simulink model "OpPointTest"  (R2024b)
settings: Solver=VariableStepAuto  StartTime=0.0  StopTime=60  FixedStep=0.02  RelTol=1e-3
values from neighbouring files (symbols this model uses):
  act_ailerons = 0    [OpPointTest_main.m]    (also in SG_model_trim.m = op.inputs(1).u; trim_op_fixed_v.mat)
  act_rear = 4    [OpPointTest_main.m]    (also in SG_model_trim.m = op.inputs(2).u; trim_op_fixed_v.mat = 2.35)
  initial_P = 0    [OpPointTest_main.m]    (also in SG_model_trim.m = op.states(4).x; trim_op_fixed_v.mat)
  initial_Pitch = -3.558    [OpPointTest_main.m]    (also in SG_model_trim.m = op.states(7).x; trim_op_fixed_v.mat = 0)
  initial_Q = 0    [OpPointTest_main.m]    (also in SG_model_trim.m = op.states(5).x; trim_op_fixed_v.mat)
  initial_R = 0    [OpPointTest_main.m]    (also in SG_model_trim.m = op.states(6).x; trim_op_fixed_v.mat)
  initial_ROLL = 0    [OpPointTest_main.m]    (also in SG_model_trim.m = op.states(8).x; trim_op_fixed_v.mat)
  initial_uspeed = cos(deg2rad(-3.558))*10.275    [OpPointTest_main.m]    (also in SG_model_trim.m = op.states(1).x; linear_model.mat = 10.285; trim_op_fixed_v.mat = 10.285)
  initial_vspeed = 0    [OpPointTest_main.m]    (also in SG_model_trim.m = op.states(2).x; trim_op_fixed_v.mat)
  initial_wspeed = sin(deg2rad(-3.558))*10.275    [OpPointTest_main.m]    (also in SG_model_trim.m = op.states(3).x; trim_op_fixed_v.mat = 0)
  initial_YAW = 0    [OpPointTest_main.m]    (also in SG_model_trim.m = op.states(9).x; trim_op_fixed_v.mat)
  initial_Z = 100    [OpPointTest_main.m]    (also in SG_model_trim.m = op.states(10).x; trim_op_fixed_v.mat = -50)
  T = 2679.2979205956    (= 2679.2979206)    [OpPointTest_main.m]    (also in SG01_Flight_Dynamics.m = rho*(Rpms_propeller/60)^2*diam^4*kt; SG01_Flight_Dynamics_original.m = rho*(Rpms_propeller/60)^2*diam^4*kt; SG_model_trim.m = op.inputs(3).u; trim_op_fixed_v.mat = 4651.4278561)
settings Model: Creator=Basile  LastModifiedBy=ricar
settings SolverCC: ConcurrentTasks=on  ZeroCrossAlgorithm=Adaptive  AlgebraicLoopSolver=TrustRegion  PositivePriorityOrder=on
settings DataIOCC: ExternalInput=getinputstruct(op_trim1)  InitialState=getstatestruct(op_trim1)  SaveOutput=off  DSMLogging=off  SaveTime=off  ReturnWorkspaceOutputs=off
settings OptimizationCC: BlockReduction=off  DefaultParameterBehavior=Inlined  UseDivisionForNetSlopeComputation=on  UseFloatMulNetSlope=on  OptimizeBlockIOStorage=off  BufferReuse=off  PassReuseOutputArgsThreshold=0  EfficientFloat2IntCast=on  OptimizeBlockOrder=speed  DifferentSizesBufferReuse=on
settings DebuggingCC: InheritedTsInSrcMsg=none  TasksWithSamePriorityMsg=none  ParameterTunabilityLossMsg=error  UniqueDataStoreMsg=error  ArithmeticOperatorsInVariantConditions=warning
settings HardwareCC: ProdBitPerLong=64  ProdLongLongMode=on  ProdHWDeviceType=Intel->x86-64 (Linux 64)
settings ModelReferenceCC: EnableRefExpFcnMdlSchedulingChecks=on
settings SFSimCC: SimUseLocalCustomCode=off  MATLABDynamicMemAlloc=off  CustomCodeUndefinedFunction=UseInterfaceOnly
settings RTWCC: Description=Simulink Real-Time  SystemTargetFile=slrealtime.tlc  TemplateMakefile=slrealtime_default_tmf  GenerateReport=on  RTWUseLocalCustomCode=off  Toolchain=Simulink Real-Time Toolchain  BuildConfiguration=Faster Runs  LaunchReport=on  CodeExecutionProfiling=on  TargetLang=C++  GPUComputeCapability=3.5  DLArmComputeVersion=19.05
settings CodeAppCC: ForceParamTrailComments=on  OperatorAnnotations=on
settings SimulinkRealTimeTargetCC: InstructionSetFMA=off  LogToMDFFile=off

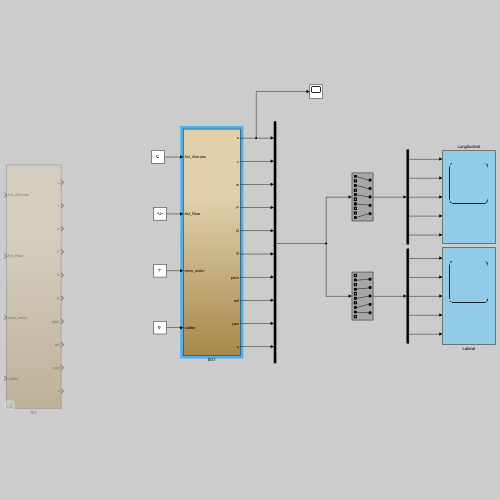
[thumbnail: Simulink's stored preview of the top-level diagram]
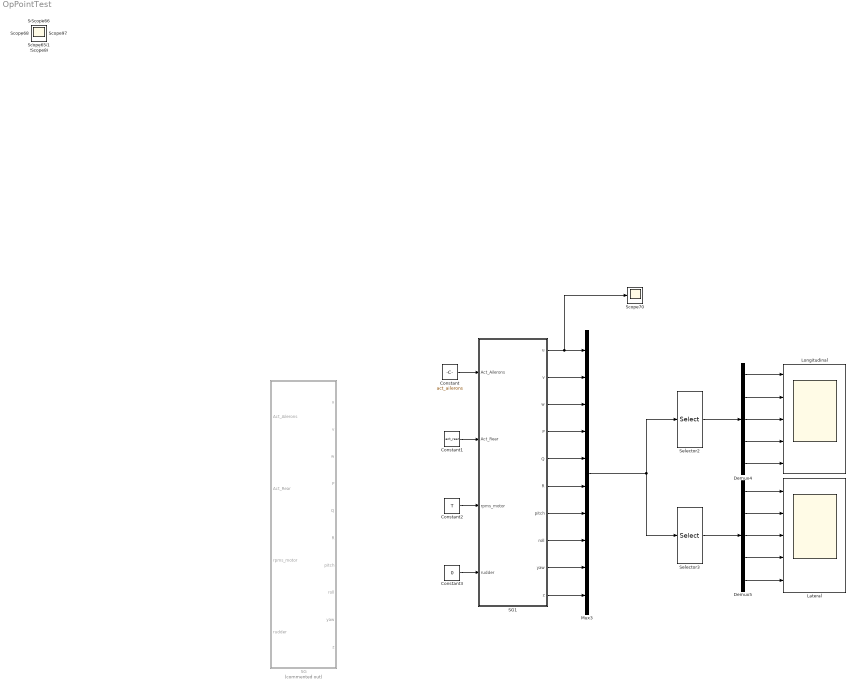
== system OpPointTest ==
  Constant : Constant  Value=act_ailerons
  Constant1 : Constant  Value=act_rear
  Constant2 : Constant  Value=T
  Constant3 : Constant  Value=0
  Demux4 : Demux  Outputs=5
  Demux5 : Demux  Outputs=5
  Lateral : Scope  NumInputPorts=5
  Longitudinal : Scope  NumInputPorts=5
  Mux3 : Mux  Inputs=10
  SG : Subsystem  Commented=on
  SG1 : Subsystem
  Scope{,1..68,70} (70 alike) : Scope
  Selector2 : Selector  InputPortWidth=10  IndexOptions=Index vector (dialog)  Indices=[1 3 5 7 10]  OutputSizes=1
  Selector3 : Selector  InputPortWidth=10  IndexOptions=Index vector (dialog)  Indices=[2 4 6 8 9]  OutputSizes=1
  wires:
  SG1/5(Q) -> Mux3/5
  SG1/6(R) -> Mux3/6
  SG1/7(pitch) -> Mux3/7
  SG1/10(z) -> Mux3/10
  SG1/4(P) -> Mux3/4
  SG1/8(roll) -> Mux3/8
  Demux5/3 -> Lateral/3
  Demux5/4 -> Lateral/4
  Selector2/1 -> Demux4/1
  Mux3/1 -> Selector2/1, Selector3/1
  Selector3/1 -> Demux5/1
  Demux5/2 -> Lateral/2
  Demux4/1 -> Longitudinal/1
  Demux5/5 -> Lateral/5
  Demux5/1 -> Lateral/1
  SG1/1(u) -> Scope70/1, Mux3/1
  SG1/9(yaw) -> Mux3/9
  Demux4/2 -> Longitudinal/2
  Demux4/4 -> Longitudinal/4
  Demux4/3 -> Longitudinal/3
  SG1/3(w) -> Mux3/3
  SG1/2(v) -> Mux3/2
  Demux4/5 -> Longitudinal/5
  Constant/1 -> SG1/1(Act_Ailerons)
  Constant1/1 -> SG1/2(Act_Rear)
  Constant2/1 -> SG1/3(rpms_motor)
  Constant3/1 -> SG1/4(rudder)

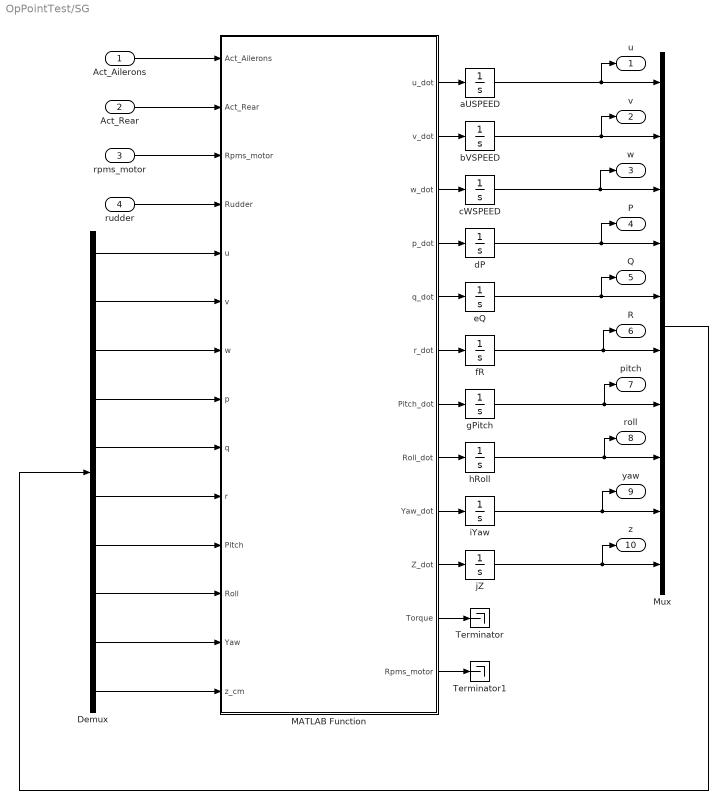
== system OpPointTest/SG ==
  Act_Ailerons : Inport
  Act_Rear : Inport  Port=2
  rpms_motor : Inport  Port=3
  rudder : Inport  Port=4
  Demux : Demux  Outputs=10
  MATLAB Function : MATLAB Function  TreatAsAtomicUnit=on
  Mux : Mux  Inputs=10
  Terminator : Terminator
  Terminator1 : Terminator
  aUSPEED : Integrator  InitialCondition=initial_uspeed
  bVSPEED : Integrator  InitialCondition=initial_vspeed
  cWSPEED : Integrator  InitialCondition=initial_wspeed
  dP : Integrator  InitialCondition=initial_P
  eQ : Integrator  InitialCondition=initial_Q
  fR : Integrator  InitialCondition=initial_R
  gPitch : Integrator  InitialCondition=initial_Pitch
  hRoll : Integrator  InitialCondition=initial_ROLL
  iYaw : Integrator  InitialCondition=initial_YAW
  jZ : Integrator  InitialCondition=initial_Z
  u : Outport
  v : Outport  Port=2
  w : Outport  Port=3
  P : Outport  Port=4
  Q : Outport  Port=5
  R : Outport  Port=6
  pitch : Outport  Port=7
  roll : Outport  Port=8
  yaw : Outport  Port=9
  z : Outport  Port=10
  wires:
  MATLAB Function/8(Roll_dot) -> hRoll/1
  Act_Rear/1 -> MATLAB Function/2(Act_Rear)
  rudder/1 -> MATLAB Function/4(Rudder)
  MATLAB Function/3(w_dot) -> cWSPEED/1
  Demux/3 -> MATLAB Function/7(w)
  MATLAB Function/11(Torque) -> Terminator/1
  MATLAB Function/6(r_dot) -> fR/1
  Demux/9 -> MATLAB Function/13(Yaw)
  Mux/1 -> Demux/1
  Demux/4 -> MATLAB Function/8(p)
  Demux/8 -> MATLAB Function/12(Roll)
  MATLAB Function/2(v_dot) -> bVSPEED/1
  Act_Ailerons/1 -> MATLAB Function/1(Act_Ailerons)
  MATLAB Function/1(u_dot) -> aUSPEED/1
  Demux/6 -> MATLAB Function/10(r)
  MATLAB Function/10(Z_dot) -> jZ/1
  rpms_motor/1 -> MATLAB Function/3("Rpms_motor ")
  MATLAB Function/12(Rpms_motor) -> Terminator1/1
  MATLAB Function/4(p_dot) -> dP/1
  Demux/1 -> MATLAB Function/5(u)
  MATLAB Function/9(Yaw_dot) -> iYaw/1
  Demux/7 -> MATLAB Function/11(Pitch)
  Demux/5 -> MATLAB Function/9(q)
  Demux/10 -> MATLAB Function/14(z_cm)
  MATLAB Function/7(Pitch_dot) -> gPitch/1
  MATLAB Function/5(q_dot) -> eQ/1
  Demux/2 -> MATLAB Function/6(v)
  aUSPEED/1 -> u/1, Mux/1
  bVSPEED/1 -> v/1, Mux/2
  cWSPEED/1 -> w/1, Mux/3
  dP/1 -> P/1, Mux/4
  eQ/1 -> Q/1, Mux/5
  fR/1 -> R/1, Mux/6
  gPitch/1 -> pitch/1, Mux/7
  hRoll/1 -> roll/1, Mux/8
  iYaw/1 -> yaw/1, Mux/9
  jZ/1 -> z/1, Mux/10

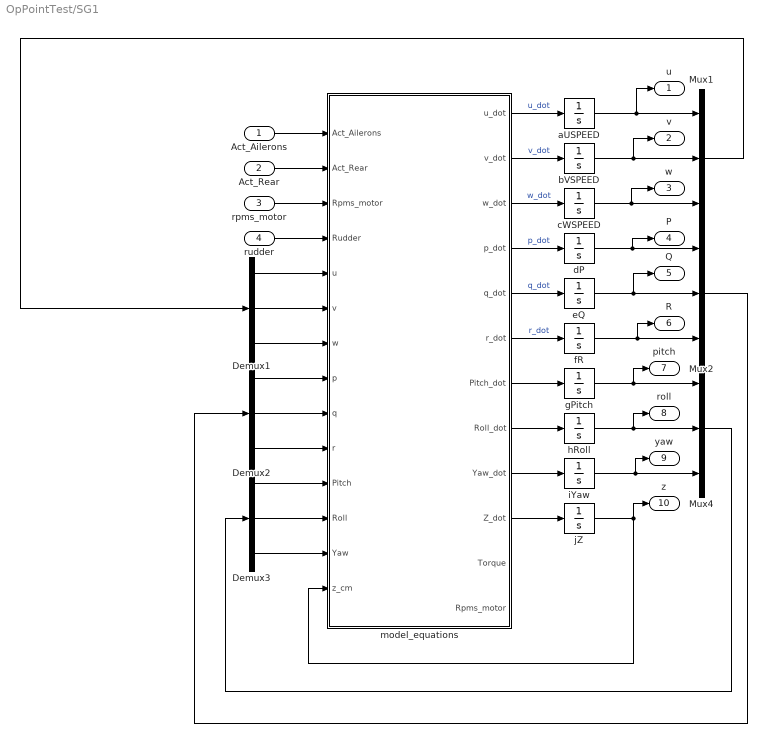
== system OpPointTest/SG1 ==
  Act_Ailerons : Inport
  Act_Rear : Inport  Port=2
  rpms_motor : Inport  Port=3
  rudder : Inport  Port=4
  Demux1 : Demux  Outputs=3
  Demux2 : Demux  Outputs=3
  Demux3 : Demux  Outputs=3
  Mux1 : Mux  Inputs=3
  Mux2 : Mux  Inputs=3
  Mux4 : Mux  Inputs=3
  aUSPEED : Integrator  InitialCondition=initial_uspeed
  bVSPEED : Integrator  InitialCondition=initial_vspeed
  cWSPEED : Integrator  InitialCondition=initial_wspeed
  dP : Integrator  InitialCondition=initial_P
  eQ : Integrator  InitialCondition=initial_Q
  fR : Integrator  InitialCondition=initial_R
  gPitch : Integrator  InitialCondition=initial_Pitch
  hRoll : Integrator  InitialCondition=initial_ROLL
  iYaw : Integrator  InitialCondition=initial_YAW
  jZ : Integrator  InitialCondition=initial_Z
  model_equations : MATLAB Function  TreatAsAtomicUnit=on  VariantControl=Variant1
  u : Outport
  v : Outport  Port=2
  w : Outport  Port=3
  P : Outport  Port=4
  Q : Outport  Port=5
  R : Outport  Port=6
  pitch : Outport  Port=7
  roll : Outport  Port=8
  yaw : Outport  Port=9
  z : Outport  Port=10
  wires:
  model_equations/3(w_dot) -> cWSPEED/1  "w_dot"
  Act_Ailerons/1 -> model_equations/1(Act_Ailerons)
  jZ/1 -> z/1, model_equations/14(z_cm)
  Mux4/1 -> Demux3/1
  model_equations/1(u_dot) -> aUSPEED/1  "u_dot"
  Demux3/1 -> model_equations/11(Pitch)
  hRoll/1 -> roll/1, Mux4/2
  model_equations/10(Z_dot) -> jZ/1
  Demux1/2 -> model_equations/6(v)
  cWSPEED/1 -> w/1, Mux1/3
  Demux1/1 -> model_equations/5(u)
  Demux1/3 -> model_equations/7(w)
  fR/1 -> R/1, Mux2/3
  Demux3/2 -> model_equations/12(Roll)
  Demux3/3 -> model_equations/13(Yaw)
  model_equations/8(Roll_dot) -> hRoll/1
  Mux2/1 -> Demux2/1
  rpms_motor/1 -> model_equations/3("Rpms_motor ")
  bVSPEED/1 -> v/1, Mux1/2
  model_equations/2(v_dot) -> bVSPEED/1  "v_dot"
  iYaw/1 -> yaw/1, Mux4/3
  aUSPEED/1 -> u/1, Mux1/1
  rudder/1 -> model_equations/4(Rudder)
  Act_Rear/1 -> model_equations/2(Act_Rear)
  model_equations/5(q_dot) -> eQ/1  "q_dot"
  Mux1/1 -> Demux1/1
  dP/1 -> Mux2/1, P/1
  eQ/1 -> Mux2/2, Q/1
  Demux2/3 -> model_equations/10(r)
  model_equations/6(r_dot) -> fR/1  "r_dot"
  gPitch/1 -> pitch/1, Mux4/1
  Demux2/1 -> model_equations/8(p)
  model_equations/9(Yaw_dot) -> iYaw/1
  model_equations/4(p_dot) -> dP/1  "p_dot"
  Demux2/2 -> model_equations/9(q)
  model_equations/7(Pitch_dot) -> gPitch/1

== matlab function OpPointTest/SG/MATLAB Function ==
  data: Act_Ailerons input; Act_Rear input; Rpms_motor input; Rudder input; u input; u_dot output; v input; w input; p input; q input; r input; Pitch input; Roll input; Yaw input; z_cm input; v_dot output; w_dot output; p_dot output; q_dot output; r_dot output; Pitch_dot output; Roll_dot output; Yaw_dot output; Z_dot output; Torque output; Rpms_motor output
function [u_dot,v_dot,w_dot,p_dot,q_dot,r_dot,Pitch_dot,Roll_dot,Yaw_dot,Z_dot,Torque,Rpms_motor] = SG01_Flight_Dynamics(Act_Ailerons,Act_Rear,Rpms_motor,Rudder,u,v,w,p,q,r,Pitch,Roll,Yaw,z_cm)

% Modelo Dinâmico do SG01, recebendo o estado do sistema ele retorna as
% derivadas das velocidades da "embarcação"

%%% CONSTANTES %%%

g = 9.81; % Gravidade (m/s^2)
rho= 1026.00; % Densidade água salgada (kg/m^3)
mu= 1.14E-3; % Coef. viscosidade dinâmica água salgada (Pa*s)
m = 2000; % Massa da "embarcação" (Kg)
Ixx = 294.2;
Iyy = 1.788e+04; % Momentos de Inércia
Izz = 1.759e+04;
Ixz = 404.7; % Produto de Inércia relevante
b = 2.400; % Span da Asa
c = 0.30988; % Corda média da Asa
S = 0.68757769; % Área da Asa
S_t = 0.20158673; % Área Elevator

wponto = 0;
struts = 1; 
if struts == 1 % struts estendidas, distancia submersa de strut
    z_struts = 1360 - z_cm/10; % estimativa muito rough
else
    z_struts = 0; % struts não estendidas INCLUIR AQUI TAMBÉM DIFERENTES DERIVADAS NO FUTURO
end


%%% DISTÂNCIAS %%% Esta secção deixou de ser necessária, acredito eu
x_cg_asas = 0.771; %centroide assumindo asa de tras semi eliptica e frente eliptica num referencial com origem a 20cm do leading edge da asa apontado para a cauda
X_CG_ASASRUDDERSTRUTS = (x_cg_asas*(S_t+S)-100*z_struts*2.825)/(S_t+S+100*z_struts); %X do CG das asa + rudder + struts no referencial com origem no meio da asa da frente CUIDADO COM O Z_STRUTS, que esta em mm
Z_CG_ASASRUDDERSTRUTS = (3*0.5*z_struts*100*z_struts)/(S_t+S+100*z_struts);
dist_CGSG_CGASAS_X = 3.715+X_CG_ASASRUDDERSTRUTS-3.964;
dist_CGSG_CGASAS_Y = 0; %idealmente
dist_CGSG_CGASAS_Z = z_struts + 1;

%%% Derivadas de estabilidade e controlo %%%
u0 = 10.285;
deltau = u - u0;
deltaAct_Rear = 2.35 - Act_Rear;
teta0 = -1.31;
Cw0 = (m*g*cos(teta0))/(0.5*rho*(u0^2)*S);
Cd1 = 0.018;

CXu = -0.03380;
CZu = -0.00166;
CMu = 0.09677;
CXa = 0.30449;
CLa = 5.65160;
CMa = -7.48898;
CXwponto = 0;
CLwponto = 0; % Não tenho como saber ainda
CMwponto = 0;
CXq = -1.10793;
CLq = 54.02705;
CMq = -344.98052;
CYb = -0.11416;
Clb = 0.10998;
CNb = 0.17299;
CYp = 0.20362;
Clp = -0.74092;
CNp = -0.42465;
CYr = 0.35551;
Clr = -0.20002;
CNr = -0.53258;
CXd_a = -0.00519;
CYd_a = 0;
CZd_a = 0.00046;
Cld_a = 0.33103;
CMd_a = 0.00124;
CNd_a = 0.02907;
CXd_t = -0.03699;
CYd_t = 0.00003;
CZd_t = -1.21190;
Cld_t = -0.00001;
CMd_t = -14.27522;
CNd_t = -0.00001;
CXd_r = -0.00023;
CYd_r = 0.09253;
CZd_r = 0.00011;
Cld_r = -0.07738;
CMd_r = 0.00146;
CNd_r = -0.14062;

%%% DERIVADAS DIMENSIONAIS DE ESTABILIDADE %%

V = sqrt(u^2 + v^2 + w^2);
beta = asin(u/V);
alpha = atan(w/V);

Xu = rho*u0*S*sin(teta0)*Cw0 + 0.5*rho*S*u0*CXu;
Zu = -rho*u0*S*cos(teta0)*Cw0 + 0.5*rho*S*u0*CZu;
Mu = 0.5*rho*S*u0*c*CMu;
du = [Xu ; Zu ; Mu];

Xw = 0.5*rho*S*u0*CXa;
CZa = -(CLa + Cd1);
Zw = 0.5*rho*S*u0*CZa;
Mw = 0.5*rho*S*u0*CMa;
dw = [Xw ; Zw ; Mw];

Xwponto = 0.25*rho*S*c*CXwponto;
CZwponto = -CLwponto;
Zwponto = 0.25*rho*S*c*CZwponto;
Mwponto = 0.25*rho*S*c*c*CMwponto;
dwponto = [Xwponto ; Zwponto ; Mwponto];

Xq = 0.25*rho*S*u0*c*CXq;
CZq = -CLq;
Zq = 0.25*rho*S*u0*c*CZq;
Mq = 0.25*rho*S*u0*c*c*CMq;
dq = [Xq ; Zq ; Mq];

Yv = 0.25*rho*S*u0*CYb;
Lv = 0.5*rho*S*u0*beta*Clb;
Nv = 0.5*rho*S*u0*beta*CNb;
dv = [Yv ; Lv ; Nv];

Yp = 0.25*rho*u0*S*beta*CYp;
Lp = 0.25*rho*u0*S*beta*beta*Clp;
Np = 0.25*rho*u0*S*beta*beta*CNp;
dp = [Yp ; Lp ; Np];

Yr = 0.25*rho*S*u0*beta*CYr;
Lr = 0.25*rho*S*u0*beta*beta*Clr;
Nr = 0.25*rho*S*u0*beta*beta*CNr;
dr = [Yr ; Lr ; Nr];

%%% DERIVADAS DIMENSIONAIS CONTRLOLO EM RADIANOS%

Act_Ailerons = deg2rad(Act_Ailerons);
Act_Rear = deg2rad(Act_Rear);
Rudder = deg2rad(Rudder);

Xd_a = 0.5*rho*u0*u0*S*CXd_a;
Yd_a = 0.5*rho*u0*u0*S*CYd_a;
Zd_a = 0.5*rho*u0*u0*S*CZd_a;
Ld_a = 0.5*rho*u0*u0*S*beta*Cld_a;
Md_a = 0.5*rho*u0*u0*S*c*CMd_a;
Nd_a = 0.5*rho*u0*u0*S*beta*CNd_a;

Xd_t = 0.5*rho*u0*u0*S*CXd_t;
Yd_t = 0.5*rho*u0*u0*S*CYd_t;
Zd_t = 0.5*rho*u0*u0*S*CZd_t;
Ld_t = 0.5*rho*u0*u0*S*beta*Cld_t;
Md_t = 0.5*rho*u0*u0*S*c*CMd_t;
Nd_t = 0.5*rho*u0*u0*S*beta*CNd_t;

Xd_r = 0.5*rho*u0*u0*S*CXd_r;
Yd_r = 0.5*rho*u0*u0*S*CYd_r;
Zd_r = 0.5*rho*u0*u0*S*CZd_r;
Ld_r = 0.5*rho*u0*u0*S*beta*Cld_r;
Md_r = 0.5*rho*u0*u0*S*c*CMd_r;
Nd_r = 0.5*rho*u0*u0*S*beta*CNd_r;

%%% ALGURES CONDIÇÃO DE VENTILAÇÃO %%%

%%% THRUST %%%

Rpms_propeller = Rpms_motor/3;
diam = 0.335;

% Coefficients for KT 
KT_p1 = -39.575462;
KT_p2 = 296.698493;
KT_p3 = -977.419765;
KT_p4 = 1855.792809;
KT_p5 = -2236.301828;
KT_p6 = 1772.128011;
KT_p7 = -922.459460;
KT_p8 = 303.597002;
KT_p9 = -57.449636;
KT_p10 = 5.069746;

% KT function 
KT = @(x) KT_p1*x.^9 + KT_p2*x.^8 + KT_p3*x.^7 + KT_p4*x.^6 + KT_p5*x.^5 + KT_p6*x.^4 + KT_p7*x.^3 + KT_p8*x.^2 + KT_p9*x + KT_p10;


% Coefficients for kq 
Kq_p1 = 2.787433;
Kq_p2 = -23.468483;
Kq_p3 = 85.725525;
Kq_p4 = -178.761944;
Kq_p5 = 234.930825;
Kq_p6 = -202.034955;
Kq_p7 = 113.775796;
Kq_p8 = -40.505237;
Kq_p9 = 8.257372;
Kq_p10 = -0.688824;

% Kq function 
Kq = @(x) Kq_p1*x.^9 + Kq_p2*x.^8 + Kq_p3*x.^7 + Kq_p4*x.^6 + Kq_p5*x.^5 + Kq_p6*x.^4 + Kq_p7*x.^3 + Kq_p8*x.^2 + Kq_p9*x + Kq_p10;


Eff_p1 = -8627.603474;
Eff_p2 = 61047.137420;
Eff_p3 = -190004.846901;
Eff_p4 = 341275.625504;
Eff_p5 = -389694.486740;
Eff_p6 = 293275.528216;
Eff_p7 = -145425.792729;
Eff_p8 = 45806.430033;
Eff_p9 = -8313.958997;
Eff_p10 = 662.693702;
% Eff function 
Eff = @(x) Eff_p1*x.^9 + Eff_p2*x.^8 + Eff_p3*x.^7 + Eff_p4*x.^6 + Eff_p5*x.^5 + Eff_p6*x.^4 + Eff_p7*x.^3 + Eff_p8*x.^2 + Eff_p9*x + Eff_p10;

js = 60*V/(Rpms_propeller*diam);

kq = Kq(js);
kt = KT(js);
eff = Eff(js);

T = rho*(Rpms_propeller/60)^2*diam^4*kt;
P_propeller = T*V/eff;

%Calculate Power usage
P_mec=P_propeller/0.8;
Torque=P_mec/(Rpms_motor*2*pi/60);

%%% SOMATÓRIO %%%

X = du(1)*deltau + dw(1)*w + dwponto(1)*wponto + dq(1)*q + Xd_a*Act_Ailerons + Xd_t*deltaAct_Rear + Xd_r*Rudder;
Y = dv(1)*v + dp(1)*p + dr(1)*r + Yd_a*Act_Ailerons + Yd_t*Act_Rear + Yd_r*Rudder;
Z = du(2)*deltau + dw(2)*w + dwponto(2)*wponto + dq(2)*q + Zd_a*Act_Ailerons + Zd_t*deltaAct_Rear + Zd_r*Rudder;
L = dv(2)*v + dp(2)*p + dr(2)*r + Ld_a*Act_Ailerons + Ld_t*Act_Rear + Ld_r*Rudder;
M = du(3)*deltau + dw(3)*w + dwponto(3)*wponto + dq(3)*q + Md_a*Act_Ailerons + Md_t*deltaAct_Rear + Md_r*Rudder;
N = dv(3)*v + dp(3)*p + dr(3)*r + Nd_a*Act_Ailerons + Nd_t*Act_Rear + Nd_r*Rudder;

%d = [dist_CGSG_CGASAS_X ; dist_CGSG_CGASAS_Y ; dist_CGSG_CGASAS_Z];
F = [X + T ; Y ; Z];
%M_1 = cross(d,F); não é necessário porque forças já estão no CG

M_2 = [L ; M ; N];

M_T = [0 ; 2.6 * T ; 0]; % Momento só do Thrust, confia

Tau = M_2 + M_T; % Momentos livres + Momentos das Forças no CG do SG


%%% DERIVADAS %%%

R = [cosd(Pitch)*cosd(Yaw) cosd(Pitch)*sind(Yaw) -sind(Pitch);
    sind(Roll)*sind(Pitch)*cosd(Yaw)-cosd(Roll)*sind(Yaw) sind(Roll)*sind(Pitch)*sind(Yaw)+cosd(Roll)*cosd(Yaw) sind(Roll)*cosd(Pitch);
    cosd(Roll)*sind(Pitch)*cosd(Yaw)+sind(Roll)*sind(Yaw) cosd(Roll)*sind(Pitch)*sind(Yaw)-sind(Roll)*cosd(Yaw) cosd(Roll)*cosd(Pitch)]; % MATRIZ DE TRANSFERÊNCIA DE REFERENCIAL

%Balance of forces
p = p*pi/180;
q = q*pi/180;
r = r*pi/180;
ww = [p;q;r];

%W_inertial = m*g*[0;0;1];
W_inertial = 0;

uvw_dot = (F + R*W_inertial)/m - cross(ww, [u;v;w]);
VI_dot = R'*[u;v;w];

%Inertial angular velocities
Q = [1 sind(Roll)*tand(Pitch) cosd(Roll)*tand(Pitch);
     0 cosd(Roll) -sind(Roll);
     0 sind(Roll)/cosd(Pitch) cosd(Roll)/cosd(Pitch)];
eul = Q*ww;
Roll_dot = eul(1);
Pitch_dot = eul(2);
Yaw_dot = eul(3);

%Balance of moments

J = [Ixx 0 Ixz;
     0   Iyy 0;
     Ixz 0 Izz];
invJ = [-Izz/(Ixz^2 - Ixx*Izz),     0,  Ixz/(Ixz^2 - Ixx*Izz);
            0,                  1/Iyy,                      0;
       Ixz/(Ixz^2 - Ixx*Izz),     0,  -Ixx/(Ixz^2 - Ixx*Izz)];

wdot = invJ*(Tau - cross(ww,J*ww));

p_dot = wdot(1)*180/pi;
q_dot = wdot(2)*180/pi;
r_dot = wdot(3)*180/pi;

u_dot = uvw_dot(1);
v_dot = uvw_dot(2);
w_dot = uvw_dot(3);

Z_dot = VI_dot(3);

% disp(Tau);
% disp(F);

% fprintf("%f %f %f %f %f %f %f %f %f %f %f %f",u_dot,v_dot,w_dot,p_dot,q_dot,r_dot,Pitch_dot,Roll_dot,Yaw_dot,Z_dot,Torque,Rpms_motor)
end

== matlab function OpPointTest/SG1/model_equations ==
  data: u_dot output; v_dot output; w_dot output; p_dot output; q_dot output; r_dot output; Pitch_dot output; Roll_dot output; Yaw_dot output; Z_dot output; Act_Ailerons input; Act_Rear input; Rpms_motor input; Rudder input; u input; v input; w input; p input; q input; r input; Pitch input; Roll input; Yaw input; Torque output; Rpms_motor output; z_cm input
function [u_dot,v_dot,w_dot,p_dot,q_dot,r_dot,Pitch_dot,Roll_dot,Yaw_dot,Z_dot,Torque,Rpms_motor] = SG01_Flight_Dynamics(Act_Ailerons,Act_Rear,Rpms_motor, Rudder,u,v,w,p,q,r,Pitch,Roll,Yaw,z_cm)

% Modelo Dinâmico do SG01, recebendo o estado do sistema ele retorna as
% derivadas das velocidades da "embarcação"

%%% CONSTANTES %%%

struts = 1;
wponto = 0;

g = 9.81; % Gravidade (m/s^2)
rho= 1026.00; % Densidade água salgada (kg/m^3)
mu= 1.14E-3; % Coef. viscosidade dinâmica água salgada (Pa*s)
m = 2000; % Massa da "embarcação" (Kg)
Ixx = 294.2;
Iyy = 1.788e+04; % Momentos de Inércia
Izz = 1.759e+04;
Ixz = 404.7; % Produto de Inércia relevante
b = 2.400; % Span da Asa
c = 0.30988; % Corda média da Asa
S = 0.68757769; % Área da Asa
S_t = 0.20158673; % Área Elevator

if struts == 1 % struts estendidas, distancia submersa de strut
    z_struts = 1360 - z_cm/10; % estimativa muito rough
else
    z_struts = 0; % struts não estendidas INCLUIR AQUI TAMBÉM DIFERENTES DERIVADAS NO FUTURO
end


%%% DISTÂNCIAS %%% Esta secção deixou de ser necessária, acredito eu
x_cg_asas = 0.771; %centroide assumindo asa de tras semi eliptica e frente eliptica num referencial com origem a 20cm do leading edge da asa apontado para a cauda
X_CG_ASASRUDDERSTRUTS = (x_cg_asas*(S_t+S)-100*z_struts*2.825)/(S_t+S+100*z_struts); %X do CG das asa + rudder + struts no referencial com origem no meio da asa da frente CUIDADO COM O Z_STRUTS, que esta em mm
Z_CG_ASASRUDDERSTRUTS = (3*0.5*z_struts*100*z_struts)/(S_t+S+100*z_struts);
dist_CGSG_CGASAS_X = 3.715+X_CG_ASASRUDDERSTRUTS-3.964;
dist_CGSG_CGASAS_Y = 0; %idealmente
dist_CGSG_CGASAS_Z = z_struts + 1;

%%% Derivadas de estabilidade e controlo %%%
V = 10.28;
u0 = cos(deg2rad(-3.558))*V;
w0 = sin(deg2rad(-3.558))*V;
deltau = u - u0;
deltaw = w - w0;
deltaAct_Rear = Act_Rear - 4;
teta0 = -3.558;
Cw0 = (m*g*cos(teta0))/(0.5*rho*(u0^2)*S);
Cd1 = 0.015;

CXu = -0.02440;
CZu = -0.00701;
CMu = 0.08341;
CXa = 0.22694;
CLa = 5.93757;
CMa = -9.37193;
CXwponto = 0;
CLwponto = 0; % Não tenho como saber ainda
CMwponto = 0;
CXq = -0.31325;
CLq = 42.62028;
CMq = -319.07598;
CYb = -0.10815;
Clb = 0.11373;
CNb = 0.15492;
CYp = 0.18263;
Clp = -0.72524;
CNp = -0.33702;
CYr = 0.32068;
Clr = -0.22191;
CNr = -0.45556;
CXd_a = -0.00673;
CYd_a = 0.02042;
CZd_a = -0.26237;
Cld_a = 0.20542;
CMd_a = 0.06255;
CNd_a = -0.01074;
CXd_t = -0.01195;
CYd_t = 0; % meti a 0 porque não faz sentido
CZd_t = -1.20579;
Cld_t = 0;
CMd_t = -13.51024;
CNd_t = 0;
CXd_r = -0.01692;
CYd_r = 0.08540;
CZd_r = -0.35782;
Cld_r = -0.19211;
CMd_r = 0.13566;
CNd_r = -0.12412;

%%% DERIVADAS DIMENSIONAIS DE ESTABILIDADE %%

beta = asin(min(u/V,1));
alpha = atan(w/V);

Xu = rho*u0*S*sin(teta0)*Cw0 + 0.5*rho*S*u0*CXu;
Zu = -rho*u0*S*cos(teta0)*Cw0 + 0.5*rho*S*u0*CZu;
Mu = 0.5*rho*S*u0*c*CMu;
du = [Xu ; Zu ; Mu];

Xw = 0.5*rho*S*u0*CXa;
CZa = -(CLa + Cd1);
Zw = 0.5*rho*S*u0*CZa;
Mw = 0.5*rho*S*u0*CMa;
dw = [Xw ; Zw ; Mw];

Xwponto = 0.25*rho*S*c*CXwponto;
CZwponto = -CLwponto;
Zwponto = 0.25*rho*S*c*CZwponto;
Mwponto = 0.25*rho*S*c*c*CMwponto;
dwponto = [Xwponto ; Zwponto ; Mwponto];

Xq = 0.25*rho*S*u0*c*CXq;
CZq = -CLq;
Zq = 0.25*rho*S*u0*c*CZq;
Mq = 0.25*rho*S*u0*c*c*CMq;
dq = [Xq ; Zq ; Mq];

Yv = 0.25*rho*S*u0*CYb;
Lv = 0.5*rho*S*u0*beta*Clb;
Nv = 0.5*rho*S*u0*beta*CNb;
dv = [Yv ; Lv ; Nv];

Yp = 0.25*rho*u0*S*beta*CYp;
Lp = 0.25*rho*u0*S*beta*beta*Clp;
Np = 0.25*rho*u0*S*beta*beta*CNp;
dp = [Yp ; Lp ; Np];

Yr = 0.25*rho*S*u0*beta*CYr;
Lr = 0.25*rho*S*u0*beta*beta*Clr;
Nr = 0.25*rho*S*u0*beta*beta*CNr;
dr = [Yr ; Lr ; Nr];

%%% DERIVADAS DIMENSIONAIS CONTRLOLO EM RADIANOS%

Act_Ailerons = deg2rad(Act_Ailerons);
Act_Rear = deg2rad(Act_Rear);
Rudder = deg2rad(Rudder);

Xd_a = 0.5*rho*u0*u0*S*CXd_a;
Yd_a = 0.5*rho*u0*u0*S*CYd_a;
Zd_a = 0.5*rho*u0*u0*S*CZd_a;
Ld_a = 0.5*rho*u0*u0*S*beta*Cld_a;
Md_a = 0.5*rho*u0*u0*S*c*CMd_a;
Nd_a = 0.5*rho*u0*u0*S*beta*CNd_a;

Xd_t = 0.5*rho*u0*u0*S*CXd_t;
Yd_t = 0.5*rho*u0*u0*S*CYd_t;
Zd_t = 0.5*rho*u0*u0*S*CZd_t;
Ld_t = 0.5*rho*u0*u0*S*beta*Cld_t;
Md_t = 0.5*rho*u0*u0*S*c*CMd_t;
Nd_t = 0.5*rho*u0*u0*S*beta*CNd_t;

Xd_r = 0.5*rho*u0*u0*S*CXd_r;
Yd_r = 0.5*rho*u0*u0*S*CYd_r;
Zd_r = 0.5*rho*u0*u0*S*CZd_r;
Ld_r = 0.5*rho*u0*u0*S*beta*Cld_r;
Md_r = 0.5*rho*u0*u0*S*c*CMd_r;
Nd_r = 0.5*rho*u0*u0*S*beta*CNd_r;

%%% ALGURES CONDIÇÃO DE VENTILAÇÃO %%%

%%% THRUST %%%

Rpms_propeller = Rpms_motor/3;
diam = 0.335;

% Coefficients for KT 
KT_p1 = -39.575;
KT_p2 = 296.698;
KT_p3 = -977.420;
KT_p4 = 1855.793;
KT_p5 = -2236.302;
KT_p6 = 1772.128;
KT_p7 = -922.459;
KT_p8 = 303.597;
KT_p9 = -57.450;
KT_p10 = 5.070;

% KT function 
KT = @(x) KT_p1*x.^9 + KT_p2*x.^8 + KT_p3*x.^7 + KT_p4*x.^6 + KT_p5*x.^5 + KT_p6*x.^4 + KT_p7*x.^3 + KT_p8*x.^2 + KT_p9*x + KT_p10;

 
% Coefficients for kq 
Kq_p1 = 2.787;
Kq_p2 = -23.468;
Kq_p3 = 85.726;
Kq_p4 = -178.762;
Kq_p5 = 234.931;
Kq_p6 = -202.035;
Kq_p7 = 113.776;
Kq_p8 = -40.505;
Kq_p9 = 8.257;
Kq_p10 = -0.689;

% Kq function 
Kq = @(x) Kq_p1*x.^9 + Kq_p2*x.^8 + Kq_p3*x.^7 + Kq_p4*x.^6 + Kq_p5*x.^5 + Kq_p6*x.^4 + Kq_p7*x.^3 + Kq_p8*x.^2 + Kq_p9*x + Kq_p10;

 
Eff_p1 = -8627.603;
Eff_p2 = 61047.137;
Eff_p3 = -190004.847;
Eff_p4 = 341275.626;
Eff_p5 = -389694.487;
Eff_p6 = 293275.528;
Eff_p7 = -145425.793;
Eff_p8 = 45806.430;
Eff_p9 = -8313.959;
Eff_p10 = 662.694;
% Eff function 
Eff = @(x) Eff_p1*x.^9 + Eff_p2*x.^8 + Eff_p3*x.^7 + Eff_p4*x.^6 + Eff_p5*x.^5 + Eff_p6*x.^4 + Eff_p7*x.^3 + Eff_p8*x.^2 + Eff_p9*x + Eff_p10;

js = 60*V/(Rpms_propeller*diam);

kq = Kq(js);
kt = KT(js);
eff = Eff(js);

T = rho*(Rpms_propeller/60)^2*diam^4*kt;
P_propeller = T*V/eff;

%Calculate Power usage
P_mec=P_propeller/0.8;
Torque=P_mec/(Rpms_motor*2*pi/60);

%%% SOMATÓRIO %%%

X = du(1)*deltau + dw(1)*deltaw + dwponto(1)*wponto + dq(1)*q + Xd_a*Act_Ailerons + Xd_t*deltaAct_Rear + Xd_r*Rudder;
Y = dv(1)*v + dp(1)*p + dr(1)*r + Yd_a*Act_Ailerons + Yd_t*Act_Rear + Yd_r*Rudder;
Z = du(2)*deltau + dw(2)*deltaw + dwponto(2)*wponto + dq(2)*q + Zd_a*Act_Ailerons + Zd_t*deltaAct_Rear + Zd_r*Rudder;
L = dv(2)*v + dp(2)*p + dr(2)*r + Ld_a*Act_Ailerons + Ld_t*Act_Rear + Ld_r*Rudder;
M = du(3)*deltau + dw(3)*deltaw + dwponto(3)*wponto + dq(3)*q + Md_a*Act_Ailerons + Md_t*deltaAct_Rear + Md_r*Rudder;
N = dv(3)*v + dp(3)*p + dr(3)*r + Nd_a*Act_Ailerons + Nd_t*Act_Rear + Nd_r*Rudder;

%d = [dist_CGSG_CGASAS_X ; dist_CGSG_CGASAS_Y ; dist_CGSG_CGASAS_Z];
F = [X + T ; Y ; Z];
%M_1 = cross(d,F); não é necessário porque forças já estão no CG

M_2 = [L ; M ; N];

M_T = [0 ; 2.6 * T; 0]; % Momento só do Thrust, confia
Tau = M_2 + M_T; % Momentos livres + Momentos das Forças no CG do SG


%%% DERIVADAS %%%

R = [cosd(Pitch)*cosd(Yaw) cosd(Pitch)*sind(Yaw) -sind(Pitch);
    sind(Roll)*sind(Pitch)*cosd(Yaw)-cosd(Roll)*sind(Yaw) sind(Roll)*sind(Pitch)*sind(Yaw)+cosd(Roll)*cosd(Yaw) sind(Roll)*cosd(Pitch);
    cosd(Roll)*sind(Pitch)*cosd(Yaw)+sind(Roll)*sind(Yaw) cosd(Roll)*sind(Pitch)*sind(Yaw)-sind(Roll)*cosd(Yaw) cosd(Roll)*cosd(Pitch)]; % MATRIZ DE TRANSFERÊNCIA DE REFERENCIAL

%Balance of forces
p = p*pi/180;
q = q*pi/180;
r = r*pi/180;
ww = [p;q;r];

%W_inertial = m*g*[0;0;1];
W_inertial = 0;

uvw_dot = (F + R*W_inertial)/m - cross(ww, [u;v;w]);
VI_dot = R'*[u;v;w];

%Inertial angular velocities
Q = [1 sind(Roll)*tand(Pitch) cosd(Roll)*tand(Pitch);
     0 cosd(Roll) -sind(Roll);
     0 sind(Roll)/cosd(Pitch) cosd(Roll)/cosd(Pitch)];
eul = Q*ww;
Roll_dot = eul(1);
Pitch_dot = eul(2);
Yaw_dot = eul(3);

%Balance of moments

J = [Ixx 0 Ixz;
     0   Iyy 0;
     Ixz 0 Izz];
invJ = [-Izz/(Ixz^2 - Ixx*Izz),     0,  Ixz/(Ixz^2 - Ixx*Izz);
            0,                  1/Iyy,                      0;
       Ixz/(Ixz^2 - Ixx*Izz),     0,  -Ixx/(Ixz^2 - Ixx*Izz)];

wdot = invJ*(Tau - cross(ww,J*ww));

p_dot = wdot(1)*180/pi;
q_dot = wdot(2)*180/pi;
r_dot = wdot(3)*180/pi;

u_dot = uvw_dot(1);
v_dot = uvw_dot(2);
w_dot = uvw_dot(3);

Z_dot = VI_dot(3);
end
